simulink model "BasicModelhost"  (Simulink 7.5)
settings: Solver=FixedStepDiscrete  StartTime=0.0  StopTime=inf  FixedStep=sp*5  RelTol=1e-3
values from neighbouring files (symbols this model uses):
  sp = 0.002    [Main.m]
undefined symbols (not defined in the file or in its folder): sfunxy_plot
libraries: xpclib x2
settings Model: Creator=Justin  LastModifiedBy=Justin
settings DataIOCC: LimitDataPoints=off  SaveOutput=off  SaveTime=off  SignalLoggingName=sigsOut
settings OptimizationCC: InlineInvariantSignals=on  InitFltsAndDblsToZero=on
settings DebuggingCC: SaveWithParameterizedLinksMsg=none  SignalResolutionControl=TryResolveAllWithWarning  SolverPrmCheckMsg=none  MultiTaskDSMMsg=warning  MultiTaskCondExecSysMsg=none  StrictBusMsg=None
settings HardwareCC: TargetUnknown=on
settings RTWCC: IncludeERTFirstTime=on
settings GRTTargetCC: TargetFcnLib=ansi_tfl_tmw.mat

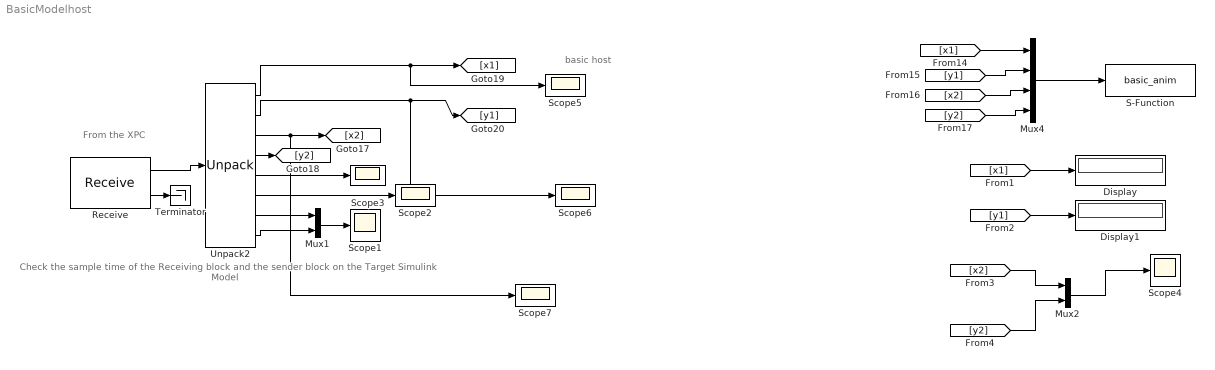
== system BasicModelhost ==
  note: From the XPC
  note: basic host
  note: Check the sample time of the Receiving block
      | and the sender block on the Target Simulink Model
  Display : Display
  Display1 : Display
  Mux1 : Mux  Inputs=2
  Mux2 : Mux  Inputs=2
  Mux4 : Mux
  Receive : xpclib/UDP/Receive  ipAddress=192.168.0.2  ipPort=25000  width=64 %32 % 8 bit for each one (i.e, two signals imply 16 bits, 3 imply 24 bits, etc.)  vblLen=off  sampletime=sp*5
  S-Function : S-Function  StartFcn=sfunxy_plot([],[],[],'Start')  StopFcn=sfunxy_plot([],[],[],'Stop')  FunctionName=basic_anim  EnableBusSupport=off
  Scope{1..7} (7 alike) : Scope
      Scope3 settings: YMin=-10  YMax=10  SaveName=ScopeData2
      Scope4 settings: YMin=-10  YMax=10  SaveName=ScopeData3
      Scope5 settings: YMin=-0.35  YMax=0.35  SaveName=ScopeData4
      Scope6 settings: SaveName=ScopeData5
      Scope7 settings: TimeRange=100  YMin=-7  YMax=6  SaveName=ScopeData6
  Terminator : Terminator
  Unpack2 : xpclib/UDP/Unpack  dimensions={1,1,1,1,1,1,1,1}  datatypes={'double','double','double','double','double','double','double','double'}  byteAlign=1
  wires:
  Receive/2 -> Terminator/1
  Receive/1 -> Unpack2/1
  [x1] -> Display/1
  [y1] -> Display1/1
  [x1] -> Mux4/1
  [y1] -> Mux4/2
  [x2] -> Mux4/3
  [y2] -> Mux4/4
  Unpack2/1 -> [x1], Scope5/1
  Unpack2/2 -> [y1], Scope6/1
  Unpack2/3 -> [x2], Scope7/1
  Unpack2/4 -> [y2]
  Mux4/1 -> S-Function/1
  Unpack2/5 -> Scope3/1
  Unpack2/6 -> Scope2/1
  Unpack2/7 -> Mux1/1
  Unpack2/8 -> Mux1/2
  Mux1/1 -> Scope1/1
  [x2] -> Mux2/1
  [y2] -> Mux2/2
  Mux2/1 -> Scope4/1
